simulink model "light_luminance_fal"  (Simulink 10.0)
settings: Solver=FixedStepAuto  StartTime=0.0  StopTime=60  FixedStep=fixedStep  MaxStep=0.2  RelTol=1e-3
undefined symbols (not defined in the file or in its folder): L0Source1, L0SourceTV, timeLightSource, timeUnauthSource
settings Model: Creator=lixuansong  LastModifiedBy=lixuansong
settings DataIOCC: SaveOutput=off  SignalLogging=off  DSMLogging=off  SaveTime=off
settings OptimizationCC: LifeSpan=auto
settings DebuggingCC: UnderspecifiedInitializationDetection=Simplified  MergeDetectMultiDrivingBlocksExec=error  SFUnexpectedBacktrackingDiag=error  SFNoUnconditionalDefaultTransitionDiag=error  SFExecutionAtInitializationDiag=warning  ArithmeticOperatorsInVariantConditions=error
settings HardwareCC: ProdBitPerPointer=64  ProdBitPerSizeT=64  ProdBitPerPtrDiffT=64  ProdLargestAtomicFloat=Float  ProdIntDivRoundTo=Zero  ProdEndianess=LittleEndian  ProdWordSize=64  ProdHWDeviceType=Intel->x86-64 (Windows64)
settings ModelReferenceCC: PropagateSignalLabelsOutOfModel=on
settings SFSimCC: SimUseLocalCustomCode=on  CustomCodeUndefinedFunction=FilterOut
settings RTWCC: RTWUseLocalCustomCode=on
settings CodeAppCC: StateflowObjectComments=off
settings GRTTargetCC: TargetLangStandard=C99 (ISO)  CombineOutputUpdateFcns=on  GRTInterface=off
settings ConfigComp: CovMetricSettings=dwe  CovHtmlReporting=off  CovSaveCumulativeToWorkspaceVar=off  CovSaveSingleToWorkspaceVar=off

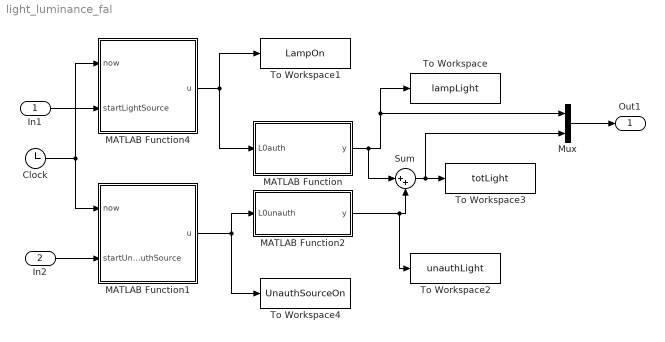
== system light_luminance_fal ==
  In1 : Inport
  In2 : Inport  Port=2
  Clock : Clock
  MATLAB Function : MATLAB Function  TreatAsAtomicUnit=on
  MATLAB Function1 : MATLAB Function  TreatAsAtomicUnit=on
  MATLAB Function2 : MATLAB Function  TreatAsAtomicUnit=on
  MATLAB Function4 : MATLAB Function  TreatAsAtomicUnit=on
  Mux : Mux  Inputs=2
  Sum : Sum  Inputs=|++
  To Workspace : ToWorkspace  VariableName=lampLight  SampleTime=-1
  To Workspace1 : ToWorkspace  VariableName=LampOn  SampleTime=-1
  To Workspace2 : ToWorkspace  VariableName=unauthLight  SampleTime=-1
  To Workspace3 : ToWorkspace  VariableName=totLight  SampleTime=-1
  To Workspace4 : ToWorkspace  VariableName=UnauthSourceOn  SampleTime=-1
  Out1 : Outport
  wires:
  MATLAB Function4/1(u) -> MATLAB Function/1(L0auth), To Workspace1/1
  Clock/1 -> MATLAB Function1/1(now), MATLAB Function4/1(now)
  MATLAB Function/1(y) -> Sum/1, Mux/1, To Workspace/1
  MATLAB Function1/1(u) -> MATLAB Function2/1(L0unauth), To Workspace4/1
  MATLAB Function2/1(y) -> To Workspace2/1, Sum/2
  Sum/1 -> Mux/2, To Workspace3/1
  In1/1 -> MATLAB Function4/2(startLightSource)
  In2/1 -> MATLAB Function1/2(startUnauthSource)
  Mux/1 -> Out1/1

== matlab function MATLAB Function1 ==
  data: u output double; now input double; timeUnauthSource parameter double; L0SourceTV parameter double; startUnauthSource input double
function u = controlLightSource2(now,timeUnauthSource,L0SourceTV, startUnauthSource)
if now>=startUnauthSource && now<=startUnauthSource+timeUnauthSource
    u=L0SourceTV;
else
    u=0;
end

== matlab function MATLAB Function ==
  data: L0auth input double; y output double; disLightSource parameter double
function y = calcLight(L0auth,disLightSource)

y=L0auth/(4*pi*disLightSource*disLightSource);

== matlab function MATLAB Function2 ==
  data: L0unauth input double; y output double; disUnauthLightSource parameter double
function y = calcUnauthLight(L0unauth, disUnauthLightSource)

y=L0unauth/(4*pi*disUnauthLightSource*disUnauthLightSource);

== matlab function MATLAB Function4 ==
  data: u output double; now input double; timeLightSource parameter double; L0Source1 parameter double; startLightSource input double
function u = controlLightSource(now,timeLightSource,L0Source1, startLightSource)
if now>=startLightSource && now<=startLightSource+timeLightSource
    u=L0Source1;
else
    u=0;
end
